simulink model "DoubleMassSimulaitonModel"  (R2022b)
settings: Solver=VariableStepAuto  StartTime=0.0  StopTime=15  MaxStep=.002  RelTol=1e-3
settings Model: Creator=hp_desktop  LastModifiedBy=hp_desktop

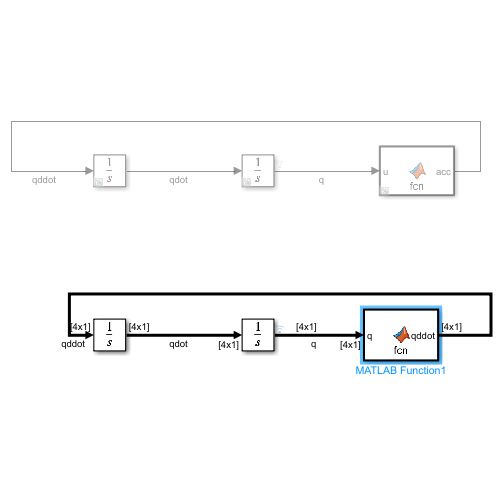
[thumbnail: Simulink's stored preview of the top-level diagram]
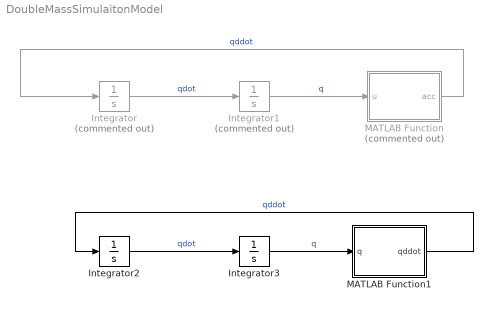
== system DoubleMassSimulaitonModel ==
  Integrator : Integrator  Commented=on  InitialCondition=[-3 -3]
  Integrator1 : Integrator  Commented=on  InitialCondition=[2, -3]
  Integrator2 : Integrator  InitialCondition=[0 0 0 0]'
  Integrator3 : Integrator  InitialCondition=[2 -3 3 0]'
  MATLAB Function : MATLAB Function  Commented=on  TreatAsAtomicUnit=on
  MATLAB Function1 : MATLAB Function  TreatAsAtomicUnit=on
  wires:
  MATLAB Function/1(acc) -> Integrator/1  "qddot"
  Integrator/1 -> Integrator1/1  "qdot"
  Integrator1/1 -> MATLAB Function/1(u)  "q"
  Integrator3/1 -> MATLAB Function1/1(q)  "q"
  Integrator2/1 -> Integrator3/1  "qdot"
  MATLAB Function1/1(qddot) -> Integrator2/1  "qddot"

== matlab function DoubleMassSimulaitonModel/MATLAB Function ==
  data: u input; acc output
function acc = fcn(u)

m = 4;
k = 3e2;
L0 = .5;
g = 9.81;


x = u(1);
y = u(2);

L = sqrt(x^2 + y^2);
cos_theta = x/L;
sin_theta = y/L;

xddot = -1/m * k *(x - L0 * cos_theta);
yddot = -1/m * (m*g + k * (y - L0 * sin_theta));

acc = [xddot, yddot];

== matlab function DoubleMassSimulaitonModel/MATLAB Function1 ==
  data: q input; qddot output
function qddot = fcn(q)

mA = 20;
mB = 8;
kA = 1e3;
kB = 2e2;
L0A = 1.2;
L0B = 1.5;
g = 9.81;


x1 = q(1);
y1 = q(2);
x2 = q(3);
y2 = q(4);


M = [...
- mA - mB,         0, -mB,   0;
      -mB,         0, -mB,   0;
        0, - mA - mB,   0, -mB;
        0,       -mB,   0, -mB];

f = [ ...

                     kA*x1*(L0A/(x1^2 + y1^2)^(1/2) - 1);
                     kB*x2*(L0B/(x2^2 + y2^2)^(1/2) - 1);
(L0A*kA*y1)/(x1^2 + y1^2)^(1/2) - g*mB - kA*y1 - g*mA;
       (L0B*kB*y2)/(x2^2 + y2^2)^(1/2) - kB*y2 - g*mB];


qddot = -M\f;
